simulink model "model"  (R2025a)
settings: Solver=VariableStepAuto  StartTime=0.0  StopTime=10.0  RelTol=1e-3
settings Model: Creator=abhi  LastModifiedBy=abhi

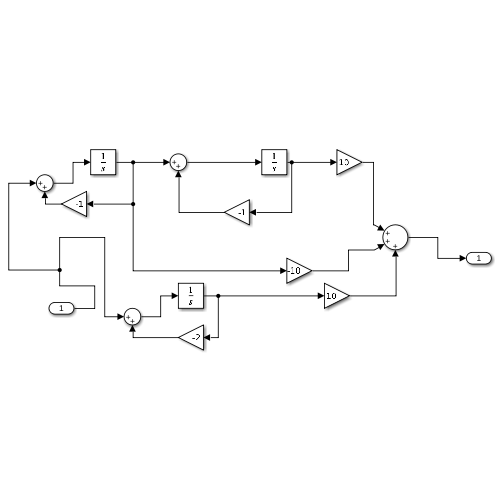
[thumbnail: Simulink's stored preview of the top-level diagram]
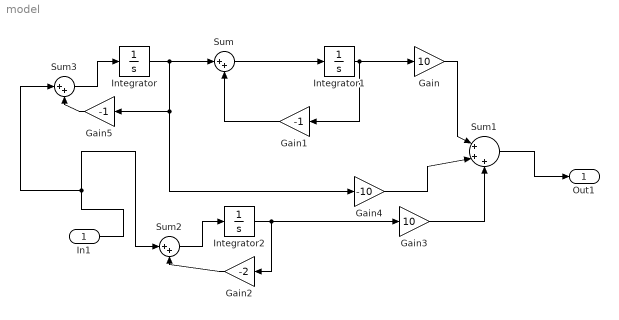
== system model ==
  In1 : Inport
  Gain : Gain  Gain=10
  Gain1 : Gain  Gain=-1
  Gain2 : Gain  Gain=-2
  Gain3 : Gain  Gain=10
  Gain4 : Gain  Gain=-10
  Gain5 : Gain  Gain=-1
  Integrator : Integrator
  Integrator1 : Integrator
  Integrator2 : Integrator
  Sum : Sum  Inputs=|++
  Sum1 : Sum  Inputs=|+++
  Sum2 : Sum  Inputs=|++
  Sum3 : Sum  Inputs=|++
  Out1 : Outport
  wires:
  Integrator/1 -> Gain5/1, Gain4/1, Sum/1
  Sum/1 -> Integrator1/1
  Integrator1/1 -> Gain1/1, Gain/1
  Gain1/1 -> Sum/2
  Gain/1 -> Sum1/1
  In1/1 -> Sum2/1, Sum3/1
  Integrator2/1 -> Gain2/1, Gain3/1
  Gain2/1 -> Sum2/2
  Sum2/1 -> Integrator2/1
  Gain3/1 -> Sum1/3
  Gain4/1 -> Sum1/2
  Gain5/1 -> Sum3/2
  Sum3/1 -> Integrator/1
  Sum1/1 -> Out1/1
